simulink model "drive_model2_2020_v2_drive_system_3"  (R2021a)
settings: Solver=VariableStepAuto  StartTime=0.0  StopTime=2  RelTol=1e-3
libraries: spsMosfetLib x6, pid_lib x5, spsSeriesRLCBranchLib x3, spsTriangleGeneratorLib x3, spsDCVoltageSourceLib x1, spsPermanentMagnetSynchronousMachineLib x1, spsThreePhaseSourceLib x1, spsUniversalBridgeLib x1, spsThreePhaseVIMeasurementLib x1, spsVoltageMeasurementLib x1, spspowerguiLib x1
settings Model: Creator=Goktug  LastModifiedBy=DELL
settings SolverCC: AlgebraicLoopSolver=TrustRegion
settings DebuggingCC: UnconnectedInputMsg=none  UnconnectedOutputMsg=none  UnconnectedLineMsg=none

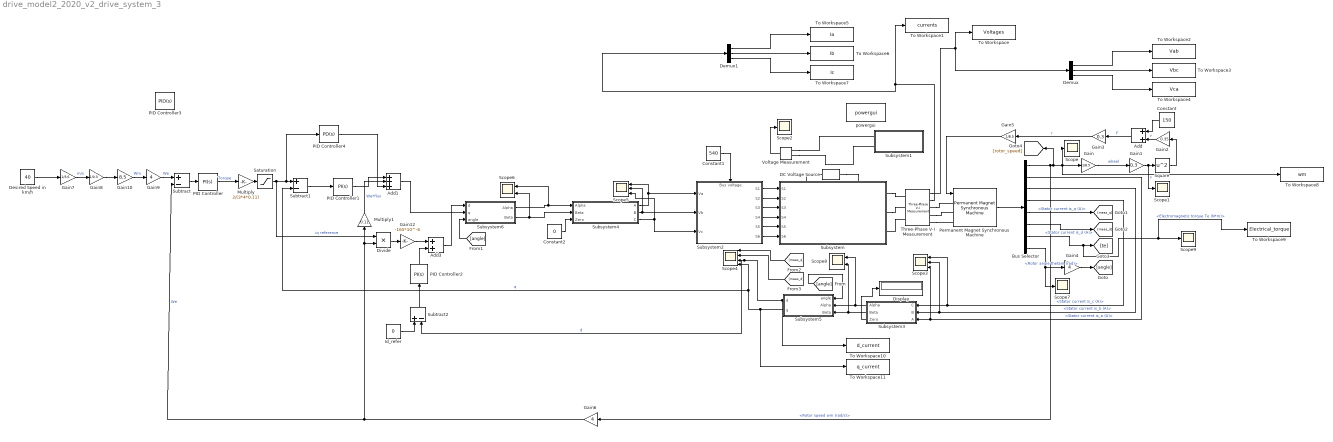
== system drive_model2_2020_v2_drive_system_3 ==
  Add : Sum
  Add1 : Sum  Inputs=+++
  Add3 : Sum
  Bus Selector : BusSelector  OutputSignals=Rotor speed wm (rad/s),Stator current is_a (A),Stator current is_b (A),Stator current is_c (A),Stator current is_q (A),Stator current is_d (A),Electromagnetic torque Te (N*m),Rotor angle thetam (rad)
  Constant : Constant  Value=150
  Constant1 : Constant  Value=540
  Constant2 : Constant  Value=0
  DC Voltage Source : spsDCVoltageSourceLib/DC Voltage Source  Amplitude=540  Measurements=None
  Demux : Demux  Outputs=3
  Demux1 : Demux  Outputs=3
  Desired Speed in km/h : Constant  Value=40
  Display : Display
  Divide : Product  Inputs=**
  Gain : Gain  Gain=1/8.5
  Gain1 : Gain  Gain=0.3
  Gain10 : Gain  Gain=8.5
  Gain12 : Gain  Gain=-165*10^-6
  Gain2 : Gain  Gain=0.35
  Gain3 : Gain  Gain=0.3
  Gain4 : Gain  Gain=4
  Gain5 : Gain  Gain=1/8.5
  Gain6 : Gain  Gain=4
  Gain7 : Gain  Gain=1/3.6
  Gain8 : Gain  Gain=1/0.3
  Gain9 : Gain  Gain=4
  Id_refer : Constant  Value=0
  Multiply : Gain  Gain=2/(3*4*0.11)
  Multiply1 : Gain  Gain=0.11
  PID Controller : pid_lib/PID Controller  Controller=PI  Form=Parallel  TimeDomain=Continuous-time  UseExternalTs=off  SampleTime=-1  IntegratorMethod=Forward Euler  FilterMethod=Forward Euler  ControllerParametersSource=internal  P=15  I=0.4  D=0  UseFilter=on  N=100  TunerSelectOption=Transfer Function Based (PID Tuner App)  InitialConditionSource=internal  InitialConditionForIntegrator=0  InitialConditionForFilter=0  DifferentiatorICPrevScaledInput=0  ExternalReset=none  TrackingMode=off  Kt=1  LimitOutput=off  SatLimitsSource=internal  UpperSaturationLimit=inf  LowerSaturationLimit=-inf  LinearizeAsGain=on  AntiWindupMode=none  Kb=1  POutMin=[]  POutMax=[]  IOutMin=[]  IOutMax=[]  DOutMin=[]  DOutMax=[]  NOutMin=[]  NOutMax=[]  SumOutMin=[]  SumOutMax=[]  SaturationOutMin=[]  SaturationOutMax=[]  PParamMin=[]  PParamMax=[]  IParamMin=[]  IParamMax=[]  DParamMin=[]  DParamMax=[]  NParamMin=[]  NParamMax=[]  KbParamMin=[]  KbParamMax=[]  KtParamMin=[]  KtParamMax=[]  KbOutMin=[]  KbOutMax=[]  KtOutMin=[]  KtOutMax=[]  IntegratorOutMin=[]  IntegratorOutMax=[]  FilterOutMin=[]  FilterOutMax=[]  SumI1OutMin=[]  SumI1OutMax=[]  SumI2OutMin=[]  SumI2OutMax=[]  SumI3OutMin=[]  SumI3OutMax=[]  SumI4OutMin=[]  SumI4OutMax=[]  SumDOutMin=[]  SumDOutMax=[]  DifferentiatorOutMin=[]  DifferentiatorOutMax=[]  FilterDiffOutCoefMin=[]  FilterDiffOutCoefMax=[]  ReciprocalOutMin=[]  ReciprocalOutMax=[]  SumDenOutMin=[]  SumDenOutMax=[]  SumNumOutMin=[]  SumNumOutMax=[]  DivideOutMin=[]  DivideOutMax=[]  UdiffTsProdOutMin=[]  UdiffTsProdOutMax=[]  NTsProdOutMin=[]  NTsProdOutMax=[]  UintegralTsProdOutMin=[]  UintegralTsProdOutMax=[]  UngainTsProdOutMin=[]  UngainTsProdOutMax=[]  IntegratorContinuousStateAttributes=''  IntegratorStateMustResolveToSignalObject=off  IntegratorRTWStateStorageClass=Auto  FilterContinuousStateAttributes=''  FilterStateMustResolveToSignalObject=off  FilterRTWStateStorageClass=Auto  ParallelPVariant=InternalParameters  IdealPVariant=Disabled  IVariant=InternalParameters  DVariant=Disabled  IntegratorVariant=Continuous  SatVariant=Disabled  AWVariant=Passthrough  PCopyVariant=Disabled  TRVariant=Disabled  FdbkBlocksVariant=Forward  IdealPFdbkVariant=Disabled  SatFdbkVariant=Disabled  DerivativeFilterVariant=Disabled  NVariant=Disabled  NCopyVariant=Disabled_SignalSpec  FilterICVariant=Disabled  IntegratorICVariant=InternalICs  ExternalResetVariant=Disabled  TRSumVariant=Passthrough  SumFdbkVariant=Disabled  SumVariant=Sum_PI  TsampFilterVariant=InternalTs  TsampNgainVariant=Passthrough  TsampIntegralVariant=Passthrough  ExternalSaturationOutDataTypeStr=Inherit: Same as second input
  PID Controller1 : pid_lib/PID Controller  Controller=PI  Form=Parallel  TimeDomain=Continuous-time  UseExternalTs=off  SampleTime=-1  IntegratorMethod=Forward Euler  FilterMethod=Forward Euler  ControllerParametersSource=internal  P=30  I=0.5  D=0  UseFilter=on  N=100  TunerSelectOption=Transfer Function Based (PID Tuner App)  InitialConditionSource=internal  InitialConditionForIntegrator=0  InitialConditionForFilter=0  DifferentiatorICPrevScaledInput=0  ExternalReset=none  TrackingMode=off  Kt=1  LimitOutput=on  SatLimitsSource=internal  UpperSaturationLimit=530  LowerSaturationLimit=-530  LinearizeAsGain=on  AntiWindupMode=clamping  Kb=1  POutMin=[]  POutMax=[]  IOutMin=-20  IOutMax=20  DOutMin=[]  DOutMax=[]  NOutMin=[]  NOutMax=[]  SumOutMin=[]  SumOutMax=[]  SaturationOutMin=[]  SaturationOutMax=[]  PParamMin=[]  PParamMax=[]  IParamMin=[]  IParamMax=[]  DParamMin=[]  DParamMax=[]  NParamMin=[]  NParamMax=[]  KbParamMin=[]  KbParamMax=[]  KtParamMin=[]  KtParamMax=[]  KbOutMin=[]  KbOutMax=[]  KtOutMin=[]  KtOutMax=[]  IntegratorOutMin=[]  IntegratorOutMax=[]  FilterOutMin=[]  FilterOutMax=[]  SumI1OutMin=[]  SumI1OutMax=[]  SumI2OutMin=[]  SumI2OutMax=[]  SumI3OutMin=[]  SumI3OutMax=[]  SumI4OutMin=[]  SumI4OutMax=[]  SumDOutMin=[]  SumDOutMax=[]  DifferentiatorOutMin=[]  DifferentiatorOutMax=[]  FilterDiffOutCoefMin=[]  FilterDiffOutCoefMax=[]  ReciprocalOutMin=[]  ReciprocalOutMax=[]  SumDenOutMin=[]  SumDenOutMax=[]  SumNumOutMin=[]  SumNumOutMax=[]  DivideOutMin=[]  DivideOutMax=[]  UdiffTsProdOutMin=[]  UdiffTsProdOutMax=[]  NTsProdOutMin=[]  NTsProdOutMax=[]  UintegralTsProdOutMin=[]  UintegralTsProdOutMax=[]  UngainTsProdOutMin=[]  UngainTsProdOutMax=[]  IntegratorContinuousStateAttributes=''  IntegratorStateMustResolveToSignalObject=off  IntegratorRTWStateStorageClass=Auto  FilterContinuousStateAttributes=''  FilterStateMustResolveToSignalObject=off  FilterRTWStateStorageClass=Auto  ParallelPVariant=InternalParameters  IdealPVariant=Disabled  IVariant=InternalParameters  DVariant=Disabled  IntegratorVariant=Continuous  SatVariant=Enabled  AWVariant=ContClampingParallel  PCopyVariant=Disabled  TRVariant=Disabled  FdbkBlocksVariant=Forward  IdealPFdbkVariant=Disabled  SatFdbkVariant=Disabled  DerivativeFilterVariant=Disabled  NVariant=Disabled  NCopyVariant=Disabled_SignalSpec  FilterICVariant=Disabled  IntegratorICVariant=InternalICs  ExternalResetVariant=Disabled  TRSumVariant=Passthrough  SumFdbkVariant=Disabled  SumVariant=Sum_PI  TsampFilterVariant=InternalTs  TsampNgainVariant=Passthrough  TsampIntegralVariant=Passthrough  ExternalSaturationOutDataTypeStr=Inherit: Same as second input
  PID Controller2 : pid_lib/PID Controller  Controller=PI  Form=Parallel  TimeDomain=Continuous-time  UseExternalTs=off  SampleTime=-1  IntegratorMethod=Forward Euler  FilterMethod=Forward Euler  ControllerParametersSource=internal  P=25  I=0.2  D=0  UseFilter=on  N=100  TunerSelectOption=Transfer Function Based (PID Tuner App)  InitialConditionSource=internal  InitialConditionForIntegrator=0  InitialConditionForFilter=0  DifferentiatorICPrevScaledInput=0  ExternalReset=none  TrackingMode=off  Kt=1  LimitOutput=off  SatLimitsSource=internal  UpperSaturationLimit=inf  LowerSaturationLimit=-inf  LinearizeAsGain=on  AntiWindupMode=none  Kb=1  POutMin=[]  POutMax=[]  IOutMin=[]  IOutMax=[]  DOutMin=[]  DOutMax=[]  NOutMin=[]  NOutMax=[]  SumOutMin=[]  SumOutMax=[]  SaturationOutMin=[]  SaturationOutMax=[]  PParamMin=[]  PParamMax=[]  IParamMin=[]  IParamMax=[]  DParamMin=[]  DParamMax=[]  NParamMin=[]  NParamMax=[]  KbParamMin=[]  KbParamMax=[]  KtParamMin=[]  KtParamMax=[]  KbOutMin=[]  KbOutMax=[]  KtOutMin=[]  KtOutMax=[]  IntegratorOutMin=[]  IntegratorOutMax=[]  FilterOutMin=[]  FilterOutMax=[]  SumI1OutMin=[]  SumI1OutMax=[]  SumI2OutMin=[]  SumI2OutMax=[]  SumI3OutMin=[]  SumI3OutMax=[]  SumI4OutMin=[]  SumI4OutMax=[]  SumDOutMin=[]  SumDOutMax=[]  DifferentiatorOutMin=[]  DifferentiatorOutMax=[]  FilterDiffOutCoefMin=[]  FilterDiffOutCoefMax=[]  ReciprocalOutMin=[]  ReciprocalOutMax=[]  SumDenOutMin=[]  SumDenOutMax=[]  SumNumOutMin=[]  SumNumOutMax=[]  DivideOutMin=[]  DivideOutMax=[]  UdiffTsProdOutMin=[]  UdiffTsProdOutMax=[]  NTsProdOutMin=[]  NTsProdOutMax=[]  UintegralTsProdOutMin=[]  UintegralTsProdOutMax=[]  UngainTsProdOutMin=[]  UngainTsProdOutMax=[]  IntegratorContinuousStateAttributes=''  IntegratorStateMustResolveToSignalObject=off  IntegratorRTWStateStorageClass=Auto  FilterContinuousStateAttributes=''  FilterStateMustResolveToSignalObject=off  FilterRTWStateStorageClass=Auto  ParallelPVariant=InternalParameters  IdealPVariant=Disabled  IVariant=InternalParameters  DVariant=Disabled  IntegratorVariant=Continuous  SatVariant=Disabled  AWVariant=Passthrough  PCopyVariant=Disabled  TRVariant=Disabled  FdbkBlocksVariant=Forward  IdealPFdbkVariant=Disabled  SatFdbkVariant=Disabled  DerivativeFilterVariant=Disabled  NVariant=Disabled  NCopyVariant=Disabled_SignalSpec  FilterICVariant=Disabled  IntegratorICVariant=InternalICs  ExternalResetVariant=Disabled  TRSumVariant=Passthrough  SumFdbkVariant=Disabled  SumVariant=Sum_PI  TsampFilterVariant=InternalTs  TsampNgainVariant=Passthrough  TsampIntegralVariant=Passthrough  ExternalSaturationOutDataTypeStr=Inherit: Same as second input
  PID Controller3 : pid_lib/PID Controller  Controller=PID  Form=Parallel  TimeDomain=Continuous-time  UseExternalTs=off  SampleTime=-1  IntegratorMethod=Forward Euler  FilterMethod=Forward Euler  ControllerParametersSource=internal  P=1  I=1  D=0  UseFilter=on  N=100  TunerSelectOption=Transfer Function Based (PID Tuner App)  InitialConditionSource=internal  InitialConditionForIntegrator=0  InitialConditionForFilter=0  DifferentiatorICPrevScaledInput=0  ExternalReset=none  TrackingMode=off  Kt=1  LimitOutput=off  SatLimitsSource=internal  UpperSaturationLimit=inf  LowerSaturationLimit=-inf  LinearizeAsGain=on  AntiWindupMode=none  Kb=1  POutMin=[]  POutMax=[]  IOutMin=[]  IOutMax=[]  DOutMin=[]  DOutMax=[]  NOutMin=[]  NOutMax=[]  SumOutMin=[]  SumOutMax=[]  SaturationOutMin=[]  SaturationOutMax=[]  PParamMin=[]  PParamMax=[]  IParamMin=[]  IParamMax=[]  DParamMin=[]  DParamMax=[]  NParamMin=[]  NParamMax=[]  KbParamMin=[]  KbParamMax=[]  KtParamMin=[]  KtParamMax=[]  KbOutMin=[]  KbOutMax=[]  KtOutMin=[]  KtOutMax=[]  IntegratorOutMin=[]  IntegratorOutMax=[]  FilterOutMin=[]  FilterOutMax=[]  SumI1OutMin=[]  SumI1OutMax=[]  SumI2OutMin=[]  SumI2OutMax=[]  SumI3OutMin=[]  SumI3OutMax=[]  SumI4OutMin=[]  SumI4OutMax=[]  SumDOutMin=[]  SumDOutMax=[]  DifferentiatorOutMin=[]  DifferentiatorOutMax=[]  FilterDiffOutCoefMin=[]  FilterDiffOutCoefMax=[]  ReciprocalOutMin=[]  ReciprocalOutMax=[]  SumDenOutMin=[]  SumDenOutMax=[]  SumNumOutMin=[]  SumNumOutMax=[]  DivideOutMin=[]  DivideOutMax=[]  UdiffTsProdOutMin=[]  UdiffTsProdOutMax=[]  NTsProdOutMin=[]  NTsProdOutMax=[]  UintegralTsProdOutMin=[]  UintegralTsProdOutMax=[]  UngainTsProdOutMin=[]  UngainTsProdOutMax=[]  IntegratorContinuousStateAttributes=''  IntegratorStateMustResolveToSignalObject=off  IntegratorRTWStateStorageClass=Auto  FilterContinuousStateAttributes=''  FilterStateMustResolveToSignalObject=off  FilterRTWStateStorageClass=Auto  ParallelPVariant=InternalParameters  IdealPVariant=Disabled  IVariant=InternalParameters  DVariant=InternalParameters  IntegratorVariant=Continuous  SatVariant=Disabled  AWVariant=Passthrough  PCopyVariant=Disabled  TRVariant=Disabled  FdbkBlocksVariant=Forward  IdealPFdbkVariant=Disabled  SatFdbkVariant=Disabled  DerivativeFilterVariant=ContFilter  NVariant=InternalParameters  NCopyVariant=Disabled  FilterICVariant=InternalICsFilter  IntegratorICVariant=InternalICs  ExternalResetVariant=Disabled  TRSumVariant=Passthrough  SumFdbkVariant=Disabled  SumVariant=Sum_PID  TsampFilterVariant=InternalTs  TsampNgainVariant=Passthrough  TsampIntegralVariant=Passthrough  ExternalSaturationOutDataTypeStr=Inherit: Same as second input
  PID Controller4 : pid_lib/PID Controller  Controller=PD  Form=Parallel  TimeDomain=Continuous-time  UseExternalTs=off  SampleTime=-1  IntegratorMethod=Forward Euler  FilterMethod=Forward Euler  ControllerParametersSource=internal  P=0.016  I=1  D=165*10^-6  UseFilter=on  N=100  TunerSelectOption=Transfer Function Based (PID Tuner App)  InitialConditionSource=internal  InitialConditionForIntegrator=0  InitialConditionForFilter=0  DifferentiatorICPrevScaledInput=0  ExternalReset=none  TrackingMode=off  Kt=1  LimitOutput=off  SatLimitsSource=internal  UpperSaturationLimit=inf  LowerSaturationLimit=-inf  LinearizeAsGain=on  AntiWindupMode=none  Kb=1  POutMin=[]  POutMax=[]  IOutMin=[]  IOutMax=[]  DOutMin=[]  DOutMax=[]  NOutMin=[]  NOutMax=[]  SumOutMin=[]  SumOutMax=[]  SaturationOutMin=[]  SaturationOutMax=[]  PParamMin=[]  PParamMax=[]  IParamMin=[]  IParamMax=[]  DParamMin=[]  DParamMax=[]  NParamMin=[]  NParamMax=[]  KbParamMin=[]  KbParamMax=[]  KtParamMin=[]  KtParamMax=[]  KbOutMin=[]  KbOutMax=[]  KtOutMin=[]  KtOutMax=[]  IntegratorOutMin=[]  IntegratorOutMax=[]  FilterOutMin=[]  FilterOutMax=[]  SumI1OutMin=[]  SumI1OutMax=[]  SumI2OutMin=[]  SumI2OutMax=[]  SumI3OutMin=[]  SumI3OutMax=[]  SumI4OutMin=[]  SumI4OutMax=[]  SumDOutMin=[]  SumDOutMax=[]  DifferentiatorOutMin=[]  DifferentiatorOutMax=[]  FilterDiffOutCoefMin=[]  FilterDiffOutCoefMax=[]  ReciprocalOutMin=[]  ReciprocalOutMax=[]  SumDenOutMin=[]  SumDenOutMax=[]  SumNumOutMin=[]  SumNumOutMax=[]  DivideOutMin=[]  DivideOutMax=[]  UdiffTsProdOutMin=[]  UdiffTsProdOutMax=[]  NTsProdOutMin=[]  NTsProdOutMax=[]  UintegralTsProdOutMin=[]  UintegralTsProdOutMax=[]  UngainTsProdOutMin=[]  UngainTsProdOutMax=[]  IntegratorContinuousStateAttributes=''  IntegratorStateMustResolveToSignalObject=off  IntegratorRTWStateStorageClass=Auto  FilterContinuousStateAttributes=''  FilterStateMustResolveToSignalObject=off  FilterRTWStateStorageClass=Auto  ParallelPVariant=InternalParameters  IdealPVariant=Disabled  IVariant=Disabled  DVariant=InternalParameters  IntegratorVariant=Disabled  SatVariant=Disabled  AWVariant=Disabled  PCopyVariant=Disabled  TRVariant=Disabled  FdbkBlocksVariant=Forward  IdealPFdbkVariant=Disabled  SatFdbkVariant=Disabled  DerivativeFilterVariant=ContFilter  NVariant=InternalParameters  NCopyVariant=Disabled  FilterICVariant=InternalICsFilter  IntegratorICVariant=Disabled  ExternalResetVariant=Disabled  TRSumVariant=Passthrough  SumFdbkVariant=Disabled  SumVariant=Sum_PD  TsampFilterVariant=InternalTs  TsampNgainVariant=Passthrough  TsampIntegralVariant=Disabled_SignalSpec  ExternalSaturationOutDataTypeStr=Inherit: Same as second input
  Permanent Magnet Synchronous Machine : spsPermanentMagnetSynchronousMachineLib/Permanent Magnet Synchronous Machine  NbPhases=3  FluxDistribution=Sinusoidal  RotorType=Round  MechanicalLoad=Torque Tm  PresetModel=No  ShowDetailedParameters=on  MeasurementBus=off  Resistance=16e-3  Inductance=8.5e-3  dqInductances=[8.5e-3,8.5e-3]  La=165e-6  MachineConstant=Flux linkage established by magnets (V.s)  Flux=0.11  VoltageCst=79.8072  TorqueCst=0.66  Flat=120  Mechanical=[0.5+(139/8.5^2) 0 4 0]  PolePairs=4  InitialConditions=[275,0, 0,0]  InitialConditions5ph=[0 0 0 0 0 0]  RefAngle=Aligned with phase A axis (original Park)  IterativeDiscreteModel=Trapezoidal non iterative  TsBlock=-1  TsPowergui=0
  Saturation : Saturate  UpperLimit=530
  Scope{,1..2,7,9} (5 alike) : Scope
  Scope3 : Scope  NumInputPorts=3
  Scope4 : Scope  NumInputPorts=4
  Scope5 : Scope  NumInputPorts=3
  Scope6 : Scope  NumInputPorts=2
  Scope8 : Scope  NumInputPorts=2
  Square : Math  Operator=square  SaturateOnIntegerOverflow=on
  Subsystem : Subsystem
      settings: PortSchema="{\"entries\":[{\"content\":{\"sides\":[{\"content\":{\"connectorIds\":[\"In1\",\"In2\",\"In3\",\"In4\",\"In5\",\"In6\"]},\"type\":\"ConnectorPlacement.EquallySpacedRectSide\",\"uuid\":\"7f4ea820-4c70-4af6-9af4-0b0f241e3ef1\"},{\"content\":{\"connectorIds\":[\"RConn1\",\"RConn2\",\"RConn3\"],\"side\":\"RIGHT\"},\"type\":\"ConnectorPlacement.EquallySpacedRectSide\",\"uuid\":\"773c8554-3ddc-44eb-9c7e-8e31c6a64932\"},{\"content\":{\"connectorIds\":[\"LConn1\",\"LConn2\"],\"side\":\"TOP\"},\"type\":\"ConnectorPlacement.EquallySpacedRectSide\",\"uuid\":\"b69331c1-3701-4f00-ae63-6be74d84d27f\"}]},\"type\":\"ConnectorPlacement.EquallySpacedConnector\",\"uuid\":\"8208b667-ecd4-4b99-b733-c445d2b47d27\"}],\"packageUris\":[\"http://schema.mathworks.com/mf0/Connector/R2020b\"],\"version\":\"1.0\"}"
      mask Display: image('$imagefile'); % Use "Edit Image" on toolstrip to change.
  Subsystem1 : Subsystem
      mask Display: image('filter.PNG'); % Use "Edit Image" on toolstrip to change.
  Subsystem2 : Subsystem
      settings: PortSchema="{\"entries\":[{\"content\":{\"sides\":[{\"content\":{\"connectorIds\":[\"In1\",\"In2\",\"In3\"]},\"type\":\"ConnectorPlacement.EquallySpacedRectSide\",\"uuid\":\"d0666ac6-1dec-4257-8954-3bbe866b6081\"},{\"content\":{\"connectorIds\":[\"Out1\",\"Out2\",\"Out3\",\"Out4\",\"Out5\",\"Out6\"],\"side\":\"RIGHT\"},\"type\":\"ConnectorPlacement.EquallySpacedRectSide\",\"uuid\":\"324de184-bd34-480c-8e8d-2175cdb653d9\"},{\"content\":{\"connectorIds\":[\"In4\"],\"side\":\"TOP\"},\"type\":\"ConnectorPlacement.EquallySpacedRectSide\",\"uuid\":\"425a65fa-c5f7-43c8-81a1-424248100921\"}]},\"type\":\"ConnectorPlacement.EquallySpacedConnector\",\"uuid\":\"bae52d76-156b-4792-bddd-053c55b94b7c\"}],\"packageUris\":[\"http://schema.mathworks.com/mf0/Connector/R2020b\"],\"version\":\"1.0\"}"
  Subsystem3 : Subsystem
      mask DialogControl Control2 Prompt: Clarke Transform
      mask Display: image('$imagefile'); % Use "Edit Image" on toolstrip to change.
  Subsystem4 : Subsystem
      mask DialogControl Control2 Prompt: Inverse Clarke Transform
      mask Display: image('$imagefile'); % Use "Edit Image" on toolstrip to change.
  Subsystem5 : Subsystem
      mask Display: image('$imagefile'); % Use "Edit Image" on toolstrip to change.
  Subsystem6 : Subsystem
      mask Display: image('$imagefile'); % Use "Edit Image" on toolstrip to change.
  Subtract : Sum  Inputs=+-
  Subtract1 : Sum  Inputs=+-
  Subtract2 : Sum  Inputs=+-
  Three-Phase V-I Measurement : spsThreePhaseVIMeasurementLib/Three-Phase V-I Measurement  VoltageMeasurement=phase-to-phase  SetLabelV=off  LabelV=Vabc  Vpu=off  VpuLL=off  CurrentMeasurement=yes  SetLabelI=off  LabelI=Iabc  Ipu=off  Pbase=100e6  Vbase=500e3  OutputType=Complex  PhasorSimulation=off  PSBequivalent=0
  To Workspace : ToWorkspace  VariableName=Voltages  SaveFormat=Timeseries  SampleTime=-1
  To Workspace1 : ToWorkspace  VariableName=currents  SaveFormat=Timeseries  SampleTime=-1
  To Workspace10 : ToWorkspace  VariableName=d_current  SaveFormat=Timeseries  SampleTime=-1
  To Workspace11 : ToWorkspace  VariableName=q_current  SaveFormat=Timeseries  SampleTime=-1
  To Workspace2 : ToWorkspace  VariableName=Vab  SaveFormat=Timeseries  SampleTime=-1
  To Workspace3 : ToWorkspace  VariableName=Vbc  SaveFormat=Timeseries  SampleTime=-1
  To Workspace4 : ToWorkspace  VariableName=Vca  SaveFormat=Timeseries  SampleTime=-1
  To Workspace5 : ToWorkspace  VariableName=Ia  SaveFormat=Timeseries  SampleTime=-1
  To Workspace6 : ToWorkspace  VariableName=Ib  SaveFormat=Timeseries  SampleTime=-1
  To Workspace7 : ToWorkspace  VariableName=Ic  SaveFormat=Timeseries  SampleTime=-1
  To Workspace8 : ToWorkspace  VariableName=wm  SaveFormat=Timeseries  SampleTime=-1
  To Workspace9 : ToWorkspace  VariableName=Electrical_torque  SaveFormat=Timeseries  SampleTime=-1
  Voltage Measurement : spsVoltageMeasurementLib/Voltage Measurement  PhasorSimulation=off  OutputType=Complex  PSBequivalent=0
  powergui : spspowerguiLib/powergui  Priority=1  SimulationMode=Discrete  SampleTime=1e-6  frequency=60  Iterations=50  frequencyindice=0  Pbase=100e6  ErrMax=1e-4  UnitsV=kV  UnitsW=MW  buscounter=0  FunctionMessages=off  echomessages=off  EnableUseOfTLC=off  CurrentSourceSwitches=off  DisableSnubberDevices=off  DisableRonSwitches=off  DisableVfSwitches=off  DisplayEquations=off  AutomaticDiscreteSolvers=off  SolverType=Tustin/Backward Euler (TBE)  Interpol=off  ExternalGateDelay=off  methode=off  Ts=100  x0status=blocks  SPID=on  SwTol=0  HookPort=off  NonlinearTolerance=1e-4  nMaxIteration=100  ContinueOnMaxIteration=off  RestoreLinks=warning  ResistiveCurrentMeasurement=off  Frange=[0:2:500]  Ylog=off  Xlog=on  ShowGrid=off  save=off  variable=ZData  structure=0  ZoomFFT=off  StartTime=0.0  cycles=1  DisplayStyle=1  fundamental=60  FreqAxis=off  MaxFrequency=1000  frequencyindicesteady=1  RmsSteady=1  display=off
  wires:
  Permanent Magnet Synchronous Machine/1 -> Bus Selector/1
  Bus Selector/1 -> Gain/1, Scope/1, To Workspace8/1, [rotor_speed], Gain6/1  "<Rotor speed wm (rad/s)>"
  Gain/1 -> Gain1/1  "wheel"
  Gain1/1 -> Scope1/1, Square/1  "v"
  Square/1 -> Gain2/1
  Gain2/1 -> Add/2  "v"
  Constant/1 -> Add/1
  Add/1 -> Gain3/1  "F"
  Subsystem2/3(S3) -> Subsystem/3(S3)
  Subsystem2/2(S2) -> Subsystem/2(S2)
  Subsystem2/4(S4) -> Subsystem/4(S4)
  Subsystem2/1(S1) -> Subsystem/1(S1)
  Subsystem2/5(S5) -> Subsystem/5(S5)
  Subsystem2/6(S6) -> Subsystem/6(S6)
  Bus Selector/2 -> Scope3/3, Subsystem3/3(A)  "<Stator current is_a (A)>"
  Constant1/1 -> Subsystem2/4(Bus voltage)
  Voltage Measurement/1 -> Scope2/1
  Subsystem4/2(B) -> Subsystem2/2(Vb), Scope5/2
  Subsystem4/3(C) -> Scope5/3, Subsystem2/3(Vc)
  Constant2/1 -> Subsystem4/3(Zero)
  Subsystem6/1(Alpha) -> Scope6/1, Subsystem4/1(Alpha)
  Subsystem6/2(Beta) -> Scope6/2, Subsystem4/2(Beta)
  Bus Selector/3 -> Scope3/2, Subsystem3/2(B)  "<Stator current is_b (A)>"
  Bus Selector/4 -> Scope3/1, Subsystem3/1(C)  "<Stator current is_c (A)>"
  Subsystem3/1(Alpha) -> Subsystem5/2(Alpha), Scope8/1
  Subsystem3/2(Beta) -> Scope8/2, Subsystem5/3(Beta)
  Bus Selector/8 -> Gain4/1, Scope7/1  "<Rotor angle thetam (rad)>"
  [angle] -> Subsystem5/1(angle)
  Bus Selector/5 -> [meas_q]  "<Stator current is_q (A)>"
  Bus Selector/6 -> [meas_d]  "<Stator current is_d (A)>"
  Bus Selector/7 -> To Workspace9/1, Scope9/1, [te]  "<Electromagnetic torque Te (N*m)>"
  [angle] -> Subsystem6/3(angle)
  Subsystem4/1(A) -> Subsystem2/1(Va), Scope5/1
  Subsystem5/1(d) -> To Workspace10/1, Subtract2/2, Scope4/3  "d"
  Subsystem5/2(q) -> To Workspace11/1, Scope4/4, Subtract1/2  "q"
  [meas_d] -> Scope4/2
  [meas_q] -> Scope4/1
  Subsystem3/3(Zero) -> Display/1
  Gain4/1 -> [angle]
  Gain3/1 -> Gain5/1  "r"
  Gain5/1 -> Permanent Magnet Synchronous Machine/1
  Gain6/1 -> Subtract/2, Divide/2, Multiply1/1  "We"
  Desired Speed in km/h/1 -> Gain7/1
  Gain7/1 -> Gain8/1  "m/s"
  Gain9/1 -> Subtract/1  "We"
  Subtract/1 -> PID Controller/1
  PID Controller/1 -> Multiply/1  "Torque"
  Multiply/1 -> Saturation/1
  PID Controller1/1 -> Add1/1
  Multiply1/1 -> Add1/2  "We*flux"
  Add1/1 -> Subsystem6/2(q)
  Id_refer/1 -> Subtract2/1
  Subtract2/1 -> PID Controller2/1
  Subtract1/1 -> PID Controller1/1
  Saturation/1 -> Subtract1/1, PID Controller4/1, Divide/1  "iq reference"
  Gain8/1 -> Gain10/1
  Gain10/1 -> Gain9/1  "Wm"
  Three-Phase V-I Measurement/1 -> Demux/1, To Workspace/1
  Demux/1 -> To Workspace2/1
  Demux/3 -> To Workspace4/1
  Demux/2 -> To Workspace3/1
  Demux1/1 -> To Workspace5/1
  Demux1/3 -> To Workspace7/1
  Demux1/2 -> To Workspace6/1
  Three-Phase V-I Measurement/2 -> To Workspace1/1, Demux1/1
  Add3/1 -> Subsystem6/1(d)
  PID Controller2/1 -> Add3/2
  Gain12/1 -> Add3/1
  PID Controller4/1 -> Add1/3
  Divide/1 -> Gain12/1
  connections:
  Voltage Measurement/LConn2 -- Subsystem1/RConn2
  Voltage Measurement/LConn1 -- Subsystem1/RConn1
  DC Voltage Source/RConn1 -- Subsystem/LConn1
  DC Voltage Source/LConn1 -- Subsystem/LConn2
  Subsystem/RConn1 -- Three-Phase V-I Measurement/LConn1
  Subsystem/RConn2 -- Three-Phase V-I Measurement/LConn2
  Three-Phase V-I Measurement/LConn3 -- Subsystem/RConn3
  Three-Phase V-I Measurement/RConn3 -- Permanent Magnet Synchronous Machine/LConn3
  Three-Phase V-I Measurement/RConn2 -- Permanent Magnet Synchronous Machine/LConn2
  Three-Phase V-I Measurement/RConn1 -- Permanent Magnet Synchronous Machine/LConn1

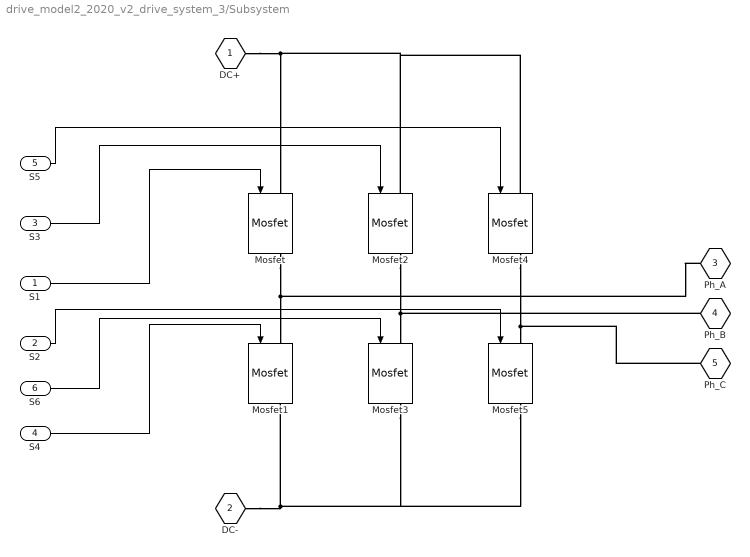
== system drive_model2_2020_v2_drive_system_3/Subsystem ==
  S1 : Inport
  S2 : Inport  Port=2
  S3 : Inport  Port=3
  S4 : Inport  Port=4
  S5 : Inport  Port=5
  S6 : Inport  Port=6
  Mosfet{,1..5} (6 alike) : spsMosfetLib/Mosfet  Ron=0.1  Lon=0  Rd=0.01  Vfd=0  IC=0  Rs=1e5  Cs=inf  Measurements=on
  DC+ : PMIOPort  Side=Left
  DC- : PMIOPort  Port=2  Side=Left
  Ph_A : PMIOPort  Port=3  Side=Right
  Ph_B : PMIOPort  Port=4  Side=Right
  Ph_C : PMIOPort  Port=5  Side=Right
  wires:
  S1/1 -> Mosfet/1
  S3/1 -> Mosfet2/1
  S5/1 -> Mosfet4/1
  S4/1 -> Mosfet1/1
  S6/1 -> Mosfet3/1
  S2/1 -> Mosfet5/1
  connections:
  Mosfet/RConn1 -- Ph_A/RConn1 -- Mosfet1/LConn1
  Mosfet2/RConn1 -- Ph_B/RConn1 -- Mosfet3/LConn1
  Mosfet4/RConn1 -- Ph_C/RConn1 -- Mosfet5/LConn1
  DC-/RConn1 -- Mosfet5/RConn1 -- Mosfet3/RConn1 -- Mosfet1/RConn1
  DC+/RConn1 -- Mosfet4/LConn1 -- Mosfet2/LConn1 -- Mosfet/LConn1

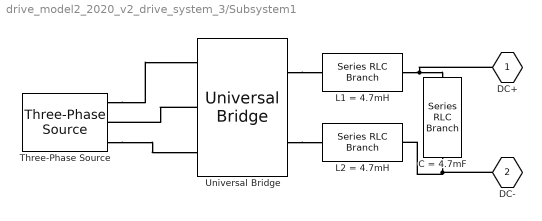
== system drive_model2_2020_v2_drive_system_3/Subsystem1 ==
  C = 4.7mF : spsSeriesRLCBranchLib/Series RLC Branch  LConnTagsString=__new0  RConnTagsString=__new0  BranchType=RC  Resistance=1e-6  Inductance=1e-3  SetiL0=off  InitialCurrent=0  Capacitance=4.7e-3  Setx0=off  InitialVoltage=0  Measurements=None
  L1 = 4.7mH : spsSeriesRLCBranchLib/Series RLC Branch  LConnTagsString=__new0  RConnTagsString=__new0  BranchType=RL  Resistance=1e-6  Inductance=4.7e-3  SetiL0=off  InitialCurrent=0  Capacitance=1e-6  Setx0=off  InitialVoltage=0  Measurements=None
  L2 = 4.7mH : spsSeriesRLCBranchLib/Series RLC Branch  LConnTagsString=__new0  RConnTagsString=__new0  BranchType=RL  Resistance=1e-6  Inductance=4.7e-3  SetiL0=off  InitialCurrent=0  Capacitance=1e-6  Setx0=off  InitialVoltage=0  Measurements=None
  Three-Phase Source : spsThreePhaseSourceLib/Three-Phase Source  InternalConnection=Yg  VoltagePhases=off  Voltage=400  PhaseAngle=0  Voltage_phases=[25e3 25e3 25e3]/sqrt(3)  PhaseAngles_phases=[0 -120 +120]  Frequency=50  NonIdealSource=off  SpecifyImpedance=off  Resistance=0.8929  Inductance=16.58e-3  ShortCircuitLevel=100e6  BaseVoltage=25e3  XRratio=7  BusType=swing  Pref=10e3  Qref=0  Prefabc=[10e3, 10e3, 10e3]  Qrefabc=[0, 0, 0]  Qmin=-inf  Qmax=inf
  Universal Bridge : spsUniversalBridgeLib/Universal Bridge  Arms=3  SnubberResistance=1e5  SnubberCapacitance=inf  Device=Diodes  Ron=1e-3  Lon=0  ForwardVoltages="[  0  0  ]"  ForwardVoltage=0  GTOparameters=[ 10e-6 , 20e-6 ]  IGBTparameters=[ 1e-6 , 2e-6 ]  Measurements=None  Measurements_2=None  converterType=Rectifier
  DC+ : PMIOPort  Side=Right
  DC- : PMIOPort  Port=2  Side=Right
  connections:
  Universal Bridge/RConn1 -- L1 = 4.7mH/LConn1
  Three-Phase Source/RConn3 -- Universal Bridge/LConn3
  C = 4.7mF/RConn1 -- DC-/RConn1 -- L2 = 4.7mH/RConn1
  Universal Bridge/RConn2 -- L2 = 4.7mH/LConn1
  Three-Phase Source/RConn1 -- Universal Bridge/LConn1
  Universal Bridge/LConn2 -- Three-Phase Source/RConn2
  L1 = 4.7mH/RConn1 -- DC+/RConn1 -- C = 4.7mF/LConn1

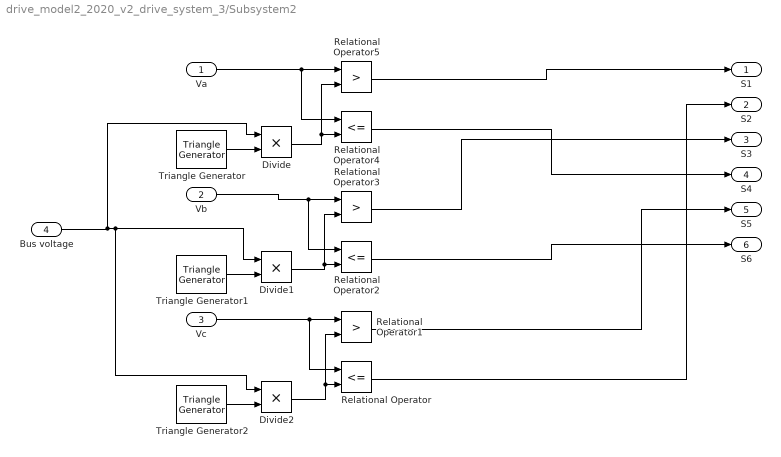
== system drive_model2_2020_v2_drive_system_3/Subsystem2 ==
  Va : Inport
  Vb : Inport  Port=2
  Vc : Inport  Port=3
  Bus voltage : Inport  Port=4
  Divide : Product  Inputs=**
  Divide1 : Product  Inputs=**
  Divide2 : Product  Inputs=**
  Relational Operator : RelationalOperator  Operator=<=  OutDataTypeStr=boolean  RndMeth=Simplest
  Relational Operator1 : RelationalOperator  Operator=>  OutDataTypeStr=boolean  RndMeth=Simplest
  Relational Operator2 : RelationalOperator  Operator=<=  OutDataTypeStr=boolean  RndMeth=Simplest
  Relational Operator3 : RelationalOperator  Operator=>  OutDataTypeStr=boolean  RndMeth=Simplest
  Relational Operator4 : RelationalOperator  Operator=<=  OutDataTypeStr=boolean  RndMeth=Simplest
  Relational Operator5 : RelationalOperator  Operator=>  OutDataTypeStr=boolean  RndMeth=Simplest
  Triangle Generator : spsTriangleGeneratorLib/Triangle Generator  Freq=10e3  Phase=0  Ts=0
  Triangle Generator1 : spsTriangleGeneratorLib/Triangle Generator  Freq=10e3  Phase=120  Ts=0
  Triangle Generator2 : spsTriangleGeneratorLib/Triangle Generator  Freq=10e3  Phase=-120  Ts=0
  S1 : Outport
  S2 : Outport  Port=2
  S3 : Outport  Port=3
  S4 : Outport  Port=4
  S5 : Outport  Port=5
  S6 : Outport  Port=6
  wires:
  Triangle Generator/1 -> Divide/2
  Triangle Generator1/1 -> Divide1/2
  Triangle Generator2/1 -> Divide2/2
  Bus voltage/1 -> Divide1/1, Divide2/1, Divide/1
  Va/1 -> Relational Operator4/1, Relational Operator5/1
  Vb/1 -> Relational Operator2/1, Relational Operator3/1
  Vc/1 -> Relational Operator/1, Relational Operator1/1
  Divide/1 -> Relational Operator4/2, Relational Operator5/2
  Divide1/1 -> Relational Operator2/2, Relational Operator3/2
  Divide2/1 -> Relational Operator/2, Relational Operator1/2
  Relational Operator5/1 -> S1/1
  Relational Operator4/1 -> S4/1
  Relational Operator3/1 -> S3/1
  Relational Operator2/1 -> S6/1
  Relational Operator1/1 -> S5/1
  Relational Operator/1 -> S2/1

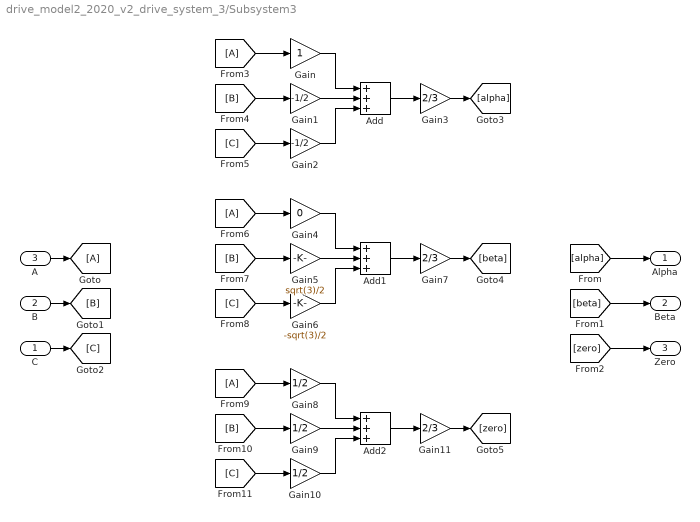
== system drive_model2_2020_v2_drive_system_3/Subsystem3 ==
  C : Inport
  B : Inport  Port=2
  A : Inport  Port=3
  Add : Sum  Inputs=+++
  Add1 : Sum  Inputs=+++
  Add2 : Sum  Inputs=+++
  Gain : Gain
  Gain1 : Gain  Gain=-1/2
  Gain10 : Gain  Gain=1/2
  Gain11 : Gain  Gain=2/3
  Gain2 : Gain  Gain=-1/2
  Gain3 : Gain  Gain=2/3
  Gain4 : Gain  Gain=0
  Gain5 : Gain  Gain=sqrt(3)/2
  Gain6 : Gain  Gain=-sqrt(3)/2
  Gain7 : Gain  Gain=2/3
  Gain8 : Gain  Gain=1/2
  Gain9 : Gain  Gain=1/2
  Alpha : Outport
  Beta : Outport  Port=2
  Zero : Outport  Port=3
  wires:
  A/1 -> [A]
  B/1 -> [B]
  C/1 -> [C]
  [alpha] -> Alpha/1
  [beta] -> Beta/1
  [zero] -> Zero/1
  Gain/1 -> Add/1
  Gain1/1 -> Add/2
  Gain2/1 -> Add/3
  Add/1 -> Gain3/1
  Gain3/1 -> [alpha]
  [C] -> Gain2/1
  [B] -> Gain1/1
  [A] -> Gain/1
  [A] -> Gain4/1
  [B] -> Gain5/1
  [C] -> Gain6/1
  Gain7/1 -> [beta]
  Add1/1 -> Gain7/1
  Gain6/1 -> Add1/3
  Gain5/1 -> Add1/2
  Gain4/1 -> Add1/1
  Gain8/1 -> Add2/1
  Gain9/1 -> Add2/2
  Gain10/1 -> Add2/3
  Add2/1 -> Gain11/1
  Gain11/1 -> [zero]
  [C] -> Gain10/1
  [B] -> Gain9/1
  [A] -> Gain8/1

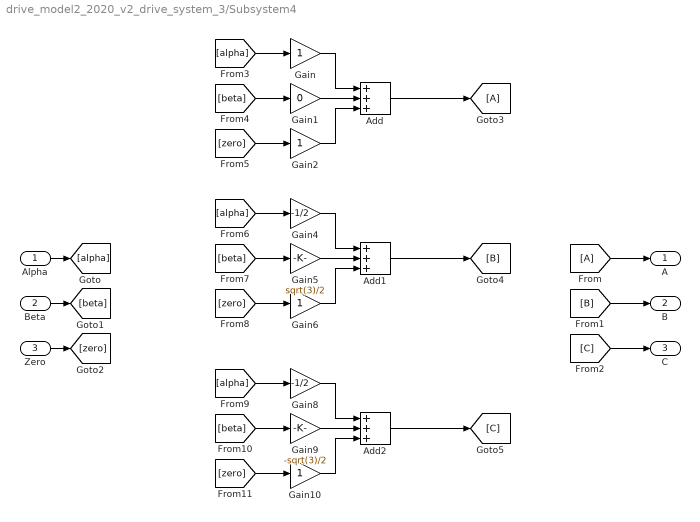
== system drive_model2_2020_v2_drive_system_3/Subsystem4 ==
  Alpha : Inport
  Beta : Inport  Port=2
  Zero : Inport  Port=3
  Add : Sum  Inputs=+++
  Add1 : Sum  Inputs=+++
  Add2 : Sum  Inputs=+++
  Gain{,2,6,10} (4 alike) : Gain
  Gain1 : Gain  Gain=0
  Gain4 : Gain  Gain=-1/2
  Gain5 : Gain  Gain=sqrt(3)/2
  Gain8 : Gain  Gain=-1/2
  Gain9 : Gain  Gain=-sqrt(3)/2
  A : Outport
  B : Outport  Port=2
  C : Outport  Port=3
  wires:
  [alpha] -> Gain8/1
  [beta] -> Gain9/1
  [zero] -> Gain10/1
  Add2/1 -> [C]
  Gain10/1 -> Add2/3
  Gain9/1 -> Add2/2
  Gain8/1 -> Add2/1
  Gain4/1 -> Add1/1
  Gain5/1 -> Add1/2
  Gain6/1 -> Add1/3
  Add1/1 -> [B]
  [zero] -> Gain6/1
  [beta] -> Gain5/1
  [alpha] -> Gain4/1
  [alpha] -> Gain/1
  [beta] -> Gain1/1
  [zero] -> Gain2/1
  Add/1 -> [A]
  Gain2/1 -> Add/3
  Gain1/1 -> Add/2
  Gain/1 -> Add/1
  [C] -> C/1
  [B] -> B/1
  [A] -> A/1
  Zero/1 -> [zero]
  Beta/1 -> [beta]
  Alpha/1 -> [alpha]

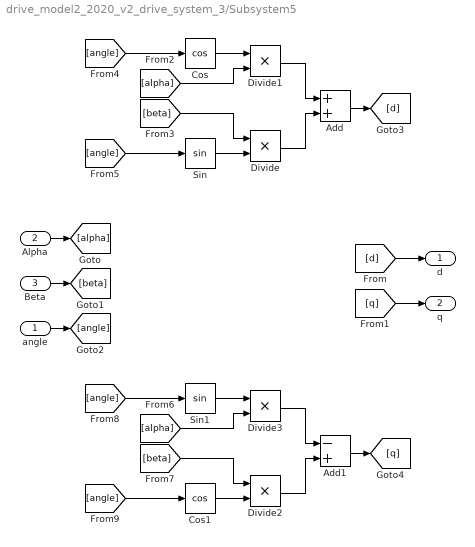
== system drive_model2_2020_v2_drive_system_3/Subsystem5 ==
  angle : Inport
  Alpha : Inport  Port=2
  Beta : Inport  Port=3
  Add : Sum
  Add1 : Sum  Inputs=-+
  Cos : Trigonometry  Operator=cos
  Cos1 : Trigonometry  Operator=cos
  Divide{,1..3} (4 alike) : Product  Inputs=**
  Sin : Trigonometry
  Sin1 : Trigonometry
  d : Outport
  q : Outport  Port=2
  wires:
  Alpha/1 -> [alpha]
  Beta/1 -> [beta]
  [q] -> q/1
  [d] -> d/1
  angle/1 -> [angle]
  Divide1/1 -> Add/1
  Divide/1 -> Add/2
  Sin/1 -> Divide/2
  Cos/1 -> Divide1/1
  [alpha] -> Divide1/2
  [beta] -> Divide/1
  [angle] -> Cos/1
  [angle] -> Sin/1
  Add/1 -> [d]
  Add1/1 -> [q]
  [beta] -> Divide2/1
  [alpha] -> Divide3/2
  Divide2/1 -> Add1/2
  Divide3/1 -> Add1/1
  [angle] -> Cos1/1
  Cos1/1 -> Divide2/2
  Sin1/1 -> Divide3/1
  [angle] -> Sin1/1

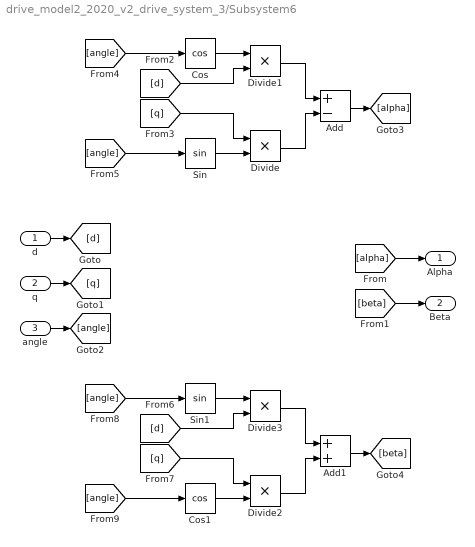
== system drive_model2_2020_v2_drive_system_3/Subsystem6 ==
  d : Inport
  q : Inport  Port=2
  angle : Inport  Port=3
  Add : Sum  Inputs=+-
  Add1 : Sum
  Cos : Trigonometry  Operator=cos
  Cos1 : Trigonometry  Operator=cos
  Divide{,1..3} (4 alike) : Product  Inputs=**
  Sin : Trigonometry
  Sin1 : Trigonometry
  Alpha : Outport
  Beta : Outport  Port=2
  wires:
  [angle] -> Sin1/1
  Sin1/1 -> Divide3/1
  Cos1/1 -> Divide2/2
  [angle] -> Cos1/1
  Divide3/1 -> Add1/1
  Divide2/1 -> Add1/2
  [d] -> Divide3/2
  [q] -> Divide2/1
  Add1/1 -> [beta]
  Add/1 -> [alpha]
  [angle] -> Sin/1
  [angle] -> Cos/1
  [q] -> Divide/1
  [d] -> Divide1/2
  Cos/1 -> Divide1/1
  Sin/1 -> Divide/2
  Divide/1 -> Add/2
  Divide1/1 -> Add/1
  angle/1 -> [angle]
  [alpha] -> Alpha/1
  [beta] -> Beta/1
  q/1 -> [q]
  d/1 -> [d]
